simulink library "RollingAliveCounter"  (R2017a)
settings: Solver=VariableStepAuto  StartTime=0.0  StopTime=10.0  RelTol=1e-3
settings Model: Creator=Di Russo  LastModifiedBy=Vraj M

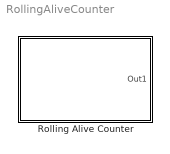
== system RollingAliveCounter ==
  Rolling Alive Counter : Subsystem

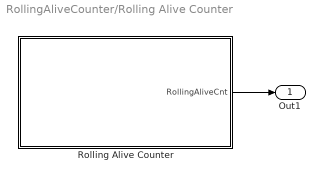
== system RollingAliveCounter/Rolling Alive Counter ==
  Rolling Alive Counter : Stateflow chart  TreatAsAtomicUnit=on
  Out1 : Outport
  wires:
  Rolling Alive Counter/1(RollingAliveCnt) -> Out1/1

== stateflow chart RollingAliveCounter/Rolling Alive Counter/Rolling Alive Counter ==
  state RollingAliveCounter
    state Count1
      en: RollingAliveCnt=0
    state Count2
      en: RollingAliveCnt=1
    state Count3
      en: RollingAliveCnt=2
    state Count4
      en: RollingAliveCnt=3
    (default) -> Count1
    Count4 -> Count1 : after(0.01,sec)
    Count1 -> Count2 : after(0.01,sec)
    Count2 -> Count3 : after(0.01,sec)
    Count3 -> Count4 : after(0.01,sec)
  data: RollingAliveCnt output double
